simulink model "allmodes"  (Simulink 7.4)
settings: Solver=ode23tb  StartTime=0.0  StopTime=inf  MaxStep=1e-4  RelTol=1e-4
undefined symbols (not defined in the file): Ion, Lithium
libraries: powerlib x185, electricdrivelib x21, powerlib_extras x19, simulink x5
(part 7 of 7)

== system allmodes/battery controller /v1/Subsystem/sawtooth generator ==
  Clock : Clock
      settings: DisableCoverage=on  Decimation=10
  Constant : Constant  DisableCoverage=on  Value=1/fsw  OutDataType=fixdt(1, 16)  OutScaling=2^0
  Divide : Product  Inputs=*/  OutDataType=fixdt(1, 16)  OutScaling=2^-10
  Gain : Gain  Gain=vc  ParameterDataType=fixdt(1, 16)  ParameterScaling=2^0  OutDataType=fixdt(1, 16)  OutScaling=2^0
  Math Function : Math  DisableCoverage=on  Operator=rem  OutDataType=fixdt(1, 16)  OutScaling=2^0  SaturateOnIntegerOverflow=on
  saw : Outport
  wires:
  Gain/1 -> saw/1
  Divide/1 -> Gain/1
  Math Function/1 -> Divide/1
  Clock/1 -> Math Function/1
  Constant/1 -> Divide/2, Math Function/2

== system allmodes/battery controller /v10/Subsystem/sawtooth generator ==
  Clock : Clock
      settings: DisableCoverage=on  Decimation=10
  Constant : Constant  DisableCoverage=on  Value=1/fsw  OutDataType=fixdt(1, 16)  OutScaling=2^0
  Divide : Product  Inputs=*/  OutDataType=fixdt(1, 16)  OutScaling=2^-10
  Gain : Gain  Gain=vc  ParameterDataType=fixdt(1, 16)  ParameterScaling=2^0  OutDataType=fixdt(1, 16)  OutScaling=2^0
  Math Function : Math  DisableCoverage=on  Operator=rem  OutDataType=fixdt(1, 16)  OutScaling=2^0  SaturateOnIntegerOverflow=on
  saw : Outport
  wires:
  Constant/1 -> Math Function/2, Divide/2
  Clock/1 -> Math Function/1
  Math Function/1 -> Divide/1
  Divide/1 -> Gain/1
  Gain/1 -> saw/1

== system allmodes/battery controller /v11/Subsystem/sawtooth generator ==
  Clock : Clock
      settings: DisableCoverage=on  Decimation=10
  Constant : Constant  DisableCoverage=on  Value=1/fsw  OutDataType=fixdt(1, 16)  OutScaling=2^0
  Divide : Product  Inputs=*/  OutDataType=fixdt(1, 16)  OutScaling=2^-10
  Gain : Gain  Gain=vc  ParameterDataType=fixdt(1, 16)  ParameterScaling=2^0  OutDataType=fixdt(1, 16)  OutScaling=2^0
  Math Function : Math  DisableCoverage=on  Operator=rem  OutDataType=fixdt(1, 16)  OutScaling=2^0  SaturateOnIntegerOverflow=on
  saw : Outport
  wires:
  Constant/1 -> Math Function/2, Divide/2
  Clock/1 -> Math Function/1
  Math Function/1 -> Divide/1
  Divide/1 -> Gain/1
  Gain/1 -> saw/1

== system allmodes/battery controller /v12/Subsystem/sawtooth generator ==
  Clock : Clock
      settings: DisableCoverage=on  Decimation=10
  Constant : Constant  DisableCoverage=on  Value=1/fsw  OutDataType=fixdt(1, 16)  OutScaling=2^0
  Divide : Product  Inputs=*/  OutDataType=fixdt(1, 16)  OutScaling=2^-10
  Gain : Gain  Gain=vc  ParameterDataType=fixdt(1, 16)  ParameterScaling=2^0  OutDataType=fixdt(1, 16)  OutScaling=2^0
  Math Function : Math  DisableCoverage=on  Operator=rem  OutDataType=fixdt(1, 16)  OutScaling=2^0  SaturateOnIntegerOverflow=on
  saw : Outport
  wires:
  Constant/1 -> Math Function/2, Divide/2
  Clock/1 -> Math Function/1
  Math Function/1 -> Divide/1
  Divide/1 -> Gain/1
  Gain/1 -> saw/1

== system allmodes/battery controller /v13/Subsystem/sawtooth generator ==
  Clock : Clock
      settings: DisableCoverage=on  Decimation=10
  Constant : Constant  DisableCoverage=on  Value=1/fsw  OutDataType=fixdt(1, 16)  OutScaling=2^0
  Divide : Product  Inputs=*/  OutDataType=fixdt(1, 16)  OutScaling=2^-10
  Gain : Gain  Gain=vc  ParameterDataType=fixdt(1, 16)  ParameterScaling=2^0  OutDataType=fixdt(1, 16)  OutScaling=2^0
  Math Function : Math  DisableCoverage=on  Operator=rem  OutDataType=fixdt(1, 16)  OutScaling=2^0  SaturateOnIntegerOverflow=on
  saw : Outport
  wires:
  Constant/1 -> Math Function/2, Divide/2
  Clock/1 -> Math Function/1
  Math Function/1 -> Divide/1
  Divide/1 -> Gain/1
  Gain/1 -> saw/1

== system allmodes/battery controller /v14/Subsystem/sawtooth generator ==
  Clock : Clock
      settings: DisableCoverage=on  Decimation=10
  Constant : Constant  DisableCoverage=on  Value=1/fsw  OutDataType=fixdt(1, 16)  OutScaling=2^0
  Divide : Product  Inputs=*/  OutDataType=fixdt(1, 16)  OutScaling=2^-10
  Gain : Gain  Gain=vc  ParameterDataType=fixdt(1, 16)  ParameterScaling=2^0  OutDataType=fixdt(1, 16)  OutScaling=2^0
  Math Function : Math  DisableCoverage=on  Operator=rem  OutDataType=fixdt(1, 16)  OutScaling=2^0  SaturateOnIntegerOverflow=on
  saw : Outport
  wires:
  Constant/1 -> Math Function/2, Divide/2
  Clock/1 -> Math Function/1
  Math Function/1 -> Divide/1
  Divide/1 -> Gain/1
  Gain/1 -> saw/1

== system allmodes/battery controller /v15/Subsystem/sawtooth generator ==
  Clock : Clock
      settings: DisableCoverage=on  Decimation=10
  Constant : Constant  DisableCoverage=on  Value=1/fsw  OutDataType=fixdt(1, 16)  OutScaling=2^0
  Divide : Product  Inputs=*/  OutDataType=fixdt(1, 16)  OutScaling=2^-10
  Gain : Gain  Gain=vc  ParameterDataType=fixdt(1, 16)  ParameterScaling=2^0  OutDataType=fixdt(1, 16)  OutScaling=2^0
  Math Function : Math  DisableCoverage=on  Operator=rem  OutDataType=fixdt(1, 16)  OutScaling=2^0  SaturateOnIntegerOverflow=on
  saw : Outport
  wires:
  Constant/1 -> Math Function/2, Divide/2
  Clock/1 -> Math Function/1
  Math Function/1 -> Divide/1
  Divide/1 -> Gain/1
  Gain/1 -> saw/1

== system allmodes/battery controller /v16/Subsystem/sawtooth generator ==
  Clock : Clock
      settings: DisableCoverage=on  Decimation=10
  Constant : Constant  DisableCoverage=on  Value=1/fsw  OutDataType=fixdt(1, 16)  OutScaling=2^0
  Divide : Product  Inputs=*/  OutDataType=fixdt(1, 16)  OutScaling=2^-10
  Gain : Gain  Gain=vc  ParameterDataType=fixdt(1, 16)  ParameterScaling=2^0  OutDataType=fixdt(1, 16)  OutScaling=2^0
  Math Function : Math  DisableCoverage=on  Operator=rem  OutDataType=fixdt(1, 16)  OutScaling=2^0  SaturateOnIntegerOverflow=on
  saw : Outport
  wires:
  Constant/1 -> Math Function/2, Divide/2
  Clock/1 -> Math Function/1
  Math Function/1 -> Divide/1
  Divide/1 -> Gain/1
  Gain/1 -> saw/1

== system allmodes/battery controller /v17/Subsystem/sawtooth generator ==
  Clock : Clock
      settings: DisableCoverage=on  Decimation=10
  Constant : Constant  DisableCoverage=on  Value=1/fsw  OutDataType=fixdt(1, 16)  OutScaling=2^0
  Divide : Product  Inputs=*/  OutDataType=fixdt(1, 16)  OutScaling=2^-10
  Gain : Gain  Gain=vc  ParameterDataType=fixdt(1, 16)  ParameterScaling=2^0  OutDataType=fixdt(1, 16)  OutScaling=2^0
  Math Function : Math  DisableCoverage=on  Operator=rem  OutDataType=fixdt(1, 16)  OutScaling=2^0  SaturateOnIntegerOverflow=on
  saw : Outport
  wires:
  Constant/1 -> Math Function/2, Divide/2
  Clock/1 -> Math Function/1
  Math Function/1 -> Divide/1
  Divide/1 -> Gain/1
  Gain/1 -> saw/1

== system allmodes/battery controller /v18/Subsystem/sawtooth generator ==
  Clock : Clock
      settings: DisableCoverage=on  Decimation=10
  Constant : Constant  DisableCoverage=on  Value=1/fsw  OutDataType=fixdt(1, 16)  OutScaling=2^0
  Divide : Product  Inputs=*/  OutDataType=fixdt(1, 16)  OutScaling=2^-10
  Gain : Gain  Gain=vc  ParameterDataType=fixdt(1, 16)  ParameterScaling=2^0  OutDataType=fixdt(1, 16)  OutScaling=2^0
  Math Function : Math  DisableCoverage=on  Operator=rem  OutDataType=fixdt(1, 16)  OutScaling=2^0  SaturateOnIntegerOverflow=on
  saw : Outport
  wires:
  Constant/1 -> Math Function/2, Divide/2
  Clock/1 -> Math Function/1
  Math Function/1 -> Divide/1
  Divide/1 -> Gain/1
  Gain/1 -> saw/1

== system allmodes/battery controller /v19/Subsystem/sawtooth generator ==
  Clock : Clock
      settings: DisableCoverage=on  Decimation=10
  Constant : Constant  DisableCoverage=on  Value=1/fsw  OutDataType=fixdt(1, 16)  OutScaling=2^0
  Divide : Product  Inputs=*/  OutDataType=fixdt(1, 16)  OutScaling=2^-10
  Gain : Gain  Gain=vc  ParameterDataType=fixdt(1, 16)  ParameterScaling=2^0  OutDataType=fixdt(1, 16)  OutScaling=2^0
  Math Function : Math  DisableCoverage=on  Operator=rem  OutDataType=fixdt(1, 16)  OutScaling=2^0  SaturateOnIntegerOverflow=on
  saw : Outport
  wires:
  Constant/1 -> Math Function/2, Divide/2
  Clock/1 -> Math Function/1
  Math Function/1 -> Divide/1
  Divide/1 -> Gain/1
  Gain/1 -> saw/1

== system allmodes/battery controller /v2/Subsystem/sawtooth generator ==
  Clock : Clock
      settings: DisableCoverage=on  Decimation=10
  Constant : Constant  DisableCoverage=on  Value=1/fsw  OutDataType=fixdt(1, 16)  OutScaling=2^0
  Divide : Product  Inputs=*/  OutDataType=fixdt(1, 16)  OutScaling=2^-10
  Gain : Gain  Gain=vc  ParameterDataType=fixdt(1, 16)  ParameterScaling=2^0  OutDataType=fixdt(1, 16)  OutScaling=2^0
  Math Function : Math  DisableCoverage=on  Operator=rem  OutDataType=fixdt(1, 16)  OutScaling=2^0  SaturateOnIntegerOverflow=on
  saw : Outport
  wires:
  Constant/1 -> Math Function/2, Divide/2
  Clock/1 -> Math Function/1
  Math Function/1 -> Divide/1
  Divide/1 -> Gain/1
  Gain/1 -> saw/1

== system allmodes/battery controller /v20/Subsystem/sawtooth generator ==
  Clock : Clock
      settings: DisableCoverage=on  Decimation=10
  Constant : Constant  DisableCoverage=on  Value=1/fsw  OutDataType=fixdt(1, 16)  OutScaling=2^0
  Divide : Product  Inputs=*/  OutDataType=fixdt(1, 16)  OutScaling=2^-10
  Gain : Gain  Gain=vc  ParameterDataType=fixdt(1, 16)  ParameterScaling=2^0  OutDataType=fixdt(1, 16)  OutScaling=2^0
  Math Function : Math  DisableCoverage=on  Operator=rem  OutDataType=fixdt(1, 16)  OutScaling=2^0  SaturateOnIntegerOverflow=on
  saw : Outport
  wires:
  Gain/1 -> saw/1
  Divide/1 -> Gain/1
  Math Function/1 -> Divide/1
  Clock/1 -> Math Function/1
  Constant/1 -> Divide/2, Math Function/2

== system allmodes/battery controller /v3/Subsystem/sawtooth generator ==
  Clock : Clock
      settings: DisableCoverage=on  Decimation=10
  Constant : Constant  DisableCoverage=on  Value=1/fsw  OutDataType=fixdt(1, 16)  OutScaling=2^0
  Divide : Product  Inputs=*/  OutDataType=fixdt(1, 16)  OutScaling=2^-10
  Gain : Gain  Gain=vc  ParameterDataType=fixdt(1, 16)  ParameterScaling=2^0  OutDataType=fixdt(1, 16)  OutScaling=2^0
  Math Function : Math  DisableCoverage=on  Operator=rem  OutDataType=fixdt(1, 16)  OutScaling=2^0  SaturateOnIntegerOverflow=on
  saw : Outport
  wires:
  Gain/1 -> saw/1
  Divide/1 -> Gain/1
  Math Function/1 -> Divide/1
  Clock/1 -> Math Function/1
  Constant/1 -> Divide/2, Math Function/2

== system allmodes/battery controller /v4/Subsystem/sawtooth generator ==
  Clock : Clock
      settings: DisableCoverage=on  Decimation=10
  Constant : Constant  DisableCoverage=on  Value=1/fsw  OutDataType=fixdt(1, 16)  OutScaling=2^0
  Divide : Product  Inputs=*/  OutDataType=fixdt(1, 16)  OutScaling=2^-10
  Gain : Gain  Gain=vc  ParameterDataType=fixdt(1, 16)  ParameterScaling=2^0  OutDataType=fixdt(1, 16)  OutScaling=2^0
  Math Function : Math  DisableCoverage=on  Operator=rem  OutDataType=fixdt(1, 16)  OutScaling=2^0  SaturateOnIntegerOverflow=on
  saw : Outport
  wires:
  Constant/1 -> Math Function/2, Divide/2
  Clock/1 -> Math Function/1
  Math Function/1 -> Divide/1
  Divide/1 -> Gain/1
  Gain/1 -> saw/1

== system allmodes/battery controller /v5/Subsystem/sawtooth generator ==
  Clock : Clock
      settings: DisableCoverage=on  Decimation=10
  Constant : Constant  DisableCoverage=on  Value=1/fsw  OutDataType=fixdt(1, 16)  OutScaling=2^0
  Divide : Product  Inputs=*/  OutDataType=fixdt(1, 16)  OutScaling=2^-10
  Gain : Gain  Gain=vc  ParameterDataType=fixdt(1, 16)  ParameterScaling=2^0  OutDataType=fixdt(1, 16)  OutScaling=2^0
  Math Function : Math  DisableCoverage=on  Operator=rem  OutDataType=fixdt(1, 16)  OutScaling=2^0  SaturateOnIntegerOverflow=on
  saw : Outport
  wires:
  Gain/1 -> saw/1
  Divide/1 -> Gain/1
  Math Function/1 -> Divide/1
  Clock/1 -> Math Function/1
  Constant/1 -> Divide/2, Math Function/2

== system allmodes/battery controller /v6/Subsystem/sawtooth generator ==
  Clock : Clock
      settings: DisableCoverage=on  Decimation=10
  Constant : Constant  DisableCoverage=on  Value=1/fsw  OutDataType=fixdt(1, 16)  OutScaling=2^0
  Divide : Product  Inputs=*/  OutDataType=fixdt(1, 16)  OutScaling=2^-10
  Gain : Gain  Gain=vc  ParameterDataType=fixdt(1, 16)  ParameterScaling=2^0  OutDataType=fixdt(1, 16)  OutScaling=2^0
  Math Function : Math  DisableCoverage=on  Operator=rem  OutDataType=fixdt(1, 16)  OutScaling=2^0  SaturateOnIntegerOverflow=on
  saw : Outport
  wires:
  Constant/1 -> Math Function/2, Divide/2
  Clock/1 -> Math Function/1
  Math Function/1 -> Divide/1
  Divide/1 -> Gain/1
  Gain/1 -> saw/1

== system allmodes/battery controller /v7/Subsystem/sawtooth generator ==
  Clock : Clock
      settings: DisableCoverage=on  Decimation=10
  Constant : Constant  DisableCoverage=on  Value=1/fsw  OutDataType=fixdt(1, 16)  OutScaling=2^0
  Divide : Product  Inputs=*/  OutDataType=fixdt(1, 16)  OutScaling=2^-10
  Gain : Gain  Gain=vc  ParameterDataType=fixdt(1, 16)  ParameterScaling=2^0  OutDataType=fixdt(1, 16)  OutScaling=2^0
  Math Function : Math  DisableCoverage=on  Operator=rem  OutDataType=fixdt(1, 16)  OutScaling=2^0  SaturateOnIntegerOverflow=on
  saw : Outport
  wires:
  Gain/1 -> saw/1
  Divide/1 -> Gain/1
  Math Function/1 -> Divide/1
  Clock/1 -> Math Function/1
  Constant/1 -> Divide/2, Math Function/2

== system allmodes/battery controller /v8/Subsystem/sawtooth generator ==
  Clock : Clock
      settings: DisableCoverage=on  Decimation=10
  Constant : Constant  DisableCoverage=on  Value=1/fsw  OutDataType=fixdt(1, 16)  OutScaling=2^0
  Divide : Product  Inputs=*/  OutDataType=fixdt(1, 16)  OutScaling=2^-10
  Gain : Gain  Gain=vc  ParameterDataType=fixdt(1, 16)  ParameterScaling=2^0  OutDataType=fixdt(1, 16)  OutScaling=2^0
  Math Function : Math  DisableCoverage=on  Operator=rem  OutDataType=fixdt(1, 16)  OutScaling=2^0  SaturateOnIntegerOverflow=on
  saw : Outport
  wires:
  Constant/1 -> Math Function/2, Divide/2
  Clock/1 -> Math Function/1
  Math Function/1 -> Divide/1
  Divide/1 -> Gain/1
  Gain/1 -> saw/1

== system allmodes/battery controller /v9/Subsystem/sawtooth generator ==
  Clock : Clock
      settings: DisableCoverage=on  Decimation=10
  Constant : Constant  DisableCoverage=on  Value=1/fsw  OutDataType=fixdt(1, 16)  OutScaling=2^0
  Divide : Product  Inputs=*/  OutDataType=fixdt(1, 16)  OutScaling=2^-10
  Gain : Gain  Gain=vc  ParameterDataType=fixdt(1, 16)  ParameterScaling=2^0  OutDataType=fixdt(1, 16)  OutScaling=2^0
  Math Function : Math  DisableCoverage=on  Operator=rem  OutDataType=fixdt(1, 16)  OutScaling=2^0  SaturateOnIntegerOverflow=on
  saw : Outport
  wires:
  Gain/1 -> saw/1
  Divide/1 -> Gain/1
  Math Function/1 -> Divide/1
  Clock/1 -> Math Function/1
  Constant/1 -> Divide/2, Math Function/2
